simulink library "INT_OilP_VD"  (R2016b)
settings: Solver=VariableStepAuto  StartTime=0.0  StopTime=10.0  RelTol=1e-3
settings Model: Creator=xinchangran  LastModifiedBy=xinchangran

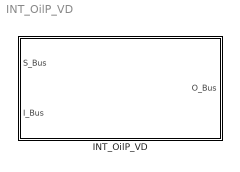
== system INT_OilP_VD ==
  INT_OilP_VD : Subsystem

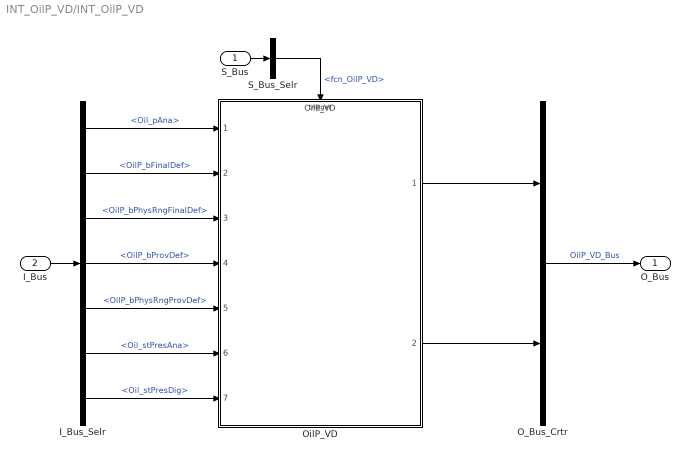
== system INT_OilP_VD/INT_OilP_VD ==
  S_Bus : Inport
  I_Bus : Inport  Port=2
  I_Bus_Selr : BusSelector  OutputSignals=Oil_pAna,OilP_bFinalDef,OilP_bPhysRngFinalDef,OilP_bProvDef,OilP_bPhysRngProvDef,Oil_stPresAna,Oil_stPresDig
  O_Bus_Crtr : BusCreator  Inputs=2
  OilP_VD : ModelReference  ModelNameDialog=OilP_VD  SimulationMode=Normal  ModelReferenceVersion=1.30  TriggerPortName=function  TriggerPortTriggerType=function-call  TriggerPortStatesWhenEnabling=held
  S_Bus_Selr : BusSelector  OutputSignals=fcn_OilP_VD
  O_Bus : Outport
  wires:
  S_Bus_Selr/1 -> OilP_VD/Trigger  "<fcn_OilP_VD>"
  S_Bus/1 -> S_Bus_Selr/1
  I_Bus/1 -> I_Bus_Selr/1
  I_Bus_Selr/1 -> OilP_VD/1  "<Oil_pAna>"
  I_Bus_Selr/2 -> OilP_VD/2  "<OilP_bFinalDef>"
  I_Bus_Selr/3 -> OilP_VD/3  "<OilP_bPhysRngFinalDef>"
  I_Bus_Selr/4 -> OilP_VD/4  "<OilP_bProvDef>"
  I_Bus_Selr/5 -> OilP_VD/5  "<OilP_bPhysRngProvDef>"
  I_Bus_Selr/6 -> OilP_VD/6  "<Oil_stPresAna>"
  I_Bus_Selr/7 -> OilP_VD/7  "<Oil_stPresDig>"
  O_Bus_Crtr/1 -> O_Bus/1  "OilP_VD_Bus"
  OilP_VD/1 -> O_Bus_Crtr/1
  OilP_VD/2 -> O_Bus_Crtr/2
